simulink model "zy7gyz1"  (R2022a)
settings: Solver=VariableStepAuto  StartTime=0.0  StopTime=50  RelTol=1e-3
settings Model: Creator=dell  LastModifiedBy=dell

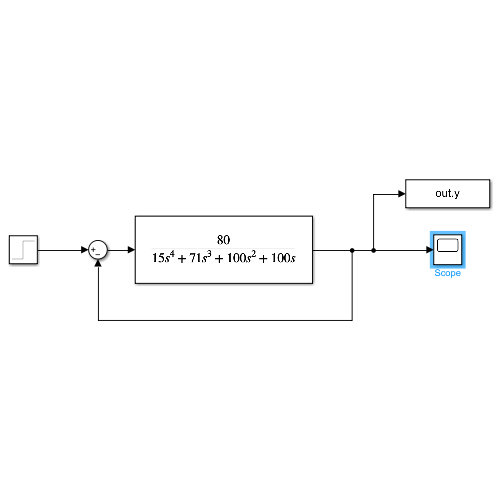
[thumbnail: Simulink's stored preview of the top-level diagram]
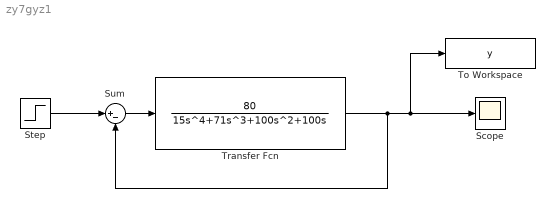
== system zy7gyz1 ==
  Scope : Scope
  Step : Step  Time=0  SampleTime=0
  Sum : Sum  Inputs=|+-
  To Workspace : ToWorkspace  VariableName=y  SaveFormat=Timeseries  SampleTime=-1
  Transfer Fcn : TransferFcn  Numerator=[80]  Denominator=[15,71,100,100,0]
  wires:
  Transfer Fcn/1 -> Sum/2, To Workspace/1, Scope/1
  Step/1 -> Sum/1
  Sum/1 -> Transfer Fcn/1
